simulink model "bldc_motor_controller_full_count"  (R2017a)
settings: Solver=FixedStepAuto  StartTime=0.0  StopTime=50000  FixedStep=1  RelTol=1e-3  EnableMultiTasking=on
libraries: simulink x10
settings Model: Creator=michael.cox4  LastModifiedBy=michael.cox4
settings OptimizationCC: DefaultParameterBehavior=Inlined  PassReuseOutputArgsAs=Individual arguments  MaxStackSize=64
settings DebuggingCC: ParameterTunabilityLossMsg=error
settings HardwareCC: ProdBitPerPointer=32  ProdBitPerSizeT=32  ProdBitPerPtrDiffT=32  ProdLargestAtomicInteger=Long  ProdLargestAtomicFloat=Double  ProdWordSize=32  ProdHWDeviceType=ARM Compatible->ARM Cortex
settings SFSimCC: MATLABDynamicMemAlloc=off
settings RTWCC: SystemTargetFile=ert.tlc  TemplateMakefile=ert_default_tmf  Description=Embedded Coder  GenerateReport=on  Toolchain=GNU Tools for ARM Embedded Processors  IncludeHyperlinkInReport=on  LaunchReport=on  GenerateTraceInfo=on  GenerateTraceReport=on  GenerateTraceReportSl=on  GenerateTraceReportSf=on  GenerateTraceReportEml=on
settings CodeAppCC: ForceParamTrailComments=on  IgnoreCustomStorageClasses=off  OperatorAnnotations=on  SimulinkDataObjDesc=on  SFDataObjDesc=on  MATLABFcnDesc=on  InsertBlockDesc=on  MATLABSourceComments=on
settings ERTTargetCC: CodeReplacementLibrary=ARM Cortex-M (Optimized)  ERTCustomFileTemplate=example_file_process.tlc

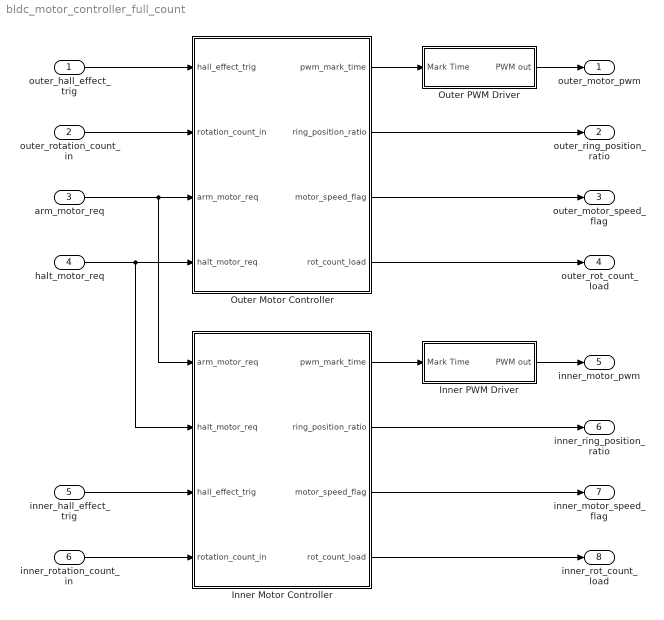
== system bldc_motor_controller_full_count ==
  outer_hall_effect_trig : Inport  OutDataTypeStr=boolean
  outer_rotation_count_in : Inport  Port=2
  arm_motor_req : Inport  Port=3
  halt_motor_req : Inport  Port=4
  inner_hall_effect_trig : Inport  Port=5  OutDataTypeStr=boolean
  inner_rotation_count_in : Inport  Port=6
  Inner Motor Controller : Subsystem
  Inner PWM Driver : Subsystem
  Outer Motor Controller : Subsystem
  Outer PWM Driver : Subsystem
  outer_motor_pwm : Outport
  outer_ring_position_ratio : Outport  Port=2
  outer_motor_speed_flag : Outport  Port=3
  outer_rot_count_load : Outport  Port=4
  inner_motor_pwm : Outport  Port=5
  inner_ring_position_ratio : Outport  Port=6
  inner_motor_speed_flag : Outport  Port=7
  inner_rot_count_load : Outport  Port=8
  wires:
  Outer Motor Controller/2(ring_position_ratio) -> outer_ring_position_ratio/1
  Outer Motor Controller/3(motor_speed_flag) -> outer_motor_speed_flag/1
  Outer PWM Driver/1(PWM out) -> outer_motor_pwm/1
  arm_motor_req/1 -> Outer Motor Controller/3(arm_motor_req), Inner Motor Controller/1(arm_motor_req)
  Outer Motor Controller/1(pwm_mark_time) -> Outer PWM Driver/1(Mark Time)
  outer_hall_effect_trig/1 -> Outer Motor Controller/1(hall_effect_trig)
  halt_motor_req/1 -> Outer Motor Controller/4(halt_motor_req), Inner Motor Controller/2(halt_motor_req)
  outer_rotation_count_in/1 -> Outer Motor Controller/2(rotation_count_in)
  Outer Motor Controller/4(rot_count_load) -> outer_rot_count_load/1
  Inner PWM Driver/1(PWM out) -> inner_motor_pwm/1
  Inner Motor Controller/4(rot_count_load) -> inner_rot_count_load/1
  Inner Motor Controller/3(motor_speed_flag) -> inner_motor_speed_flag/1
  Inner Motor Controller/2(ring_position_ratio) -> inner_ring_position_ratio/1
  Inner Motor Controller/1(pwm_mark_time) -> Inner PWM Driver/1(Mark Time)
  inner_rotation_count_in/1 -> Inner Motor Controller/4(rotation_count_in)
  inner_hall_effect_trig/1 -> Inner Motor Controller/3(hall_effect_trig)

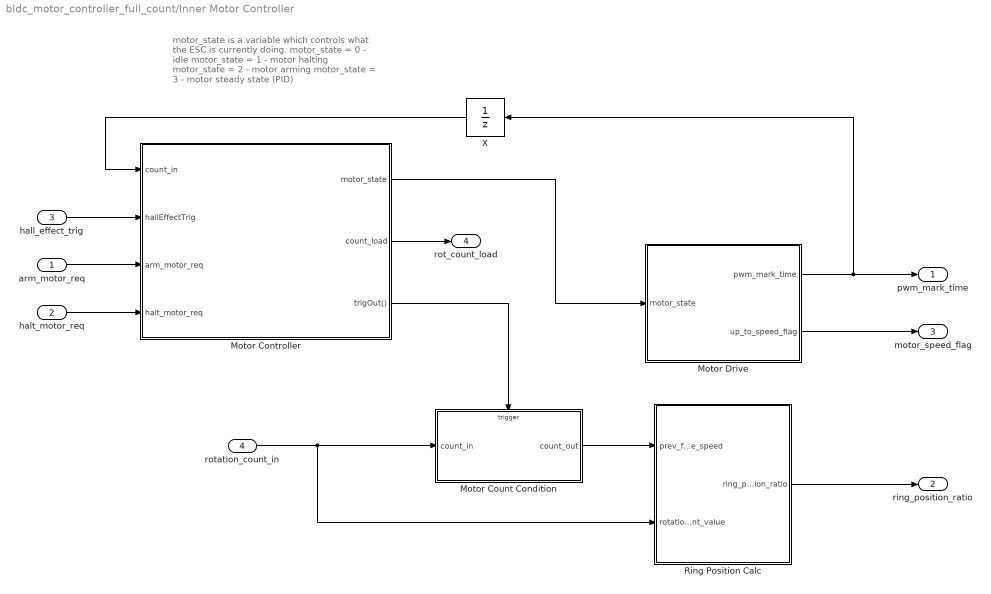
== system bldc_motor_controller_full_count/Inner Motor Controller ==
  note: motor_state is a variable which controls
      | what the ESC is currently doing.
      |   motor_state = 0 - idle
      |   motor_state = 1 - motor halting
      |   motor_state = 2 - motor arming
      |   motor_state = 3 - motor steady state (PID)
  arm_motor_req : Inport  OutDataTypeStr=boolean
  halt_motor_req : Inport  Port=2  OutDataTypeStr=boolean
  hall_effect_trig : Inport  Port=3  OutDataTypeStr=boolean
  rotation_count_in : Inport  Port=4
  Motor Controller : Stateflow chart  TreatAsAtomicUnit=on
  Motor Count Condition : Subsystem  TreatAsAtomicUnit=on
  Motor Drive : Subsystem
  Ring Position Calc : Subsystem
  X : UnitDelay  SampleTime=-1  StateName=X
  pwm_mark_time : Outport
  ring_position_ratio : Outport  Port=2
  motor_speed_flag : Outport  Port=3
  rot_count_load : Outport  Port=4
  wires:
  Motor Controller/3(trigOut()) -> Motor Count Condition/Trigger
  Motor Controller/2(count_load) -> rot_count_load/1
  Motor Count Condition/1(count_out) -> Ring Position Calc/1(prev_frame_speed)
  rotation_count_in/1 -> Motor Count Condition/1(count_in), Ring Position Calc/2(rotation_count_value)
  Motor Controller/1(motor_state) -> Motor Drive/1(motor_state)
  arm_motor_req/1 -> Motor Controller/3(arm_motor_req)
  halt_motor_req/1 -> Motor Controller/4(halt_motor_req)
  Ring Position Calc/1(ring_position_ratio) -> ring_position_ratio/1
  Motor Drive/1(pwm_mark_time) -> X/1, pwm_mark_time/1
  hall_effect_trig/1 -> Motor Controller/2(hallEffectTrig)
  X/1 -> Motor Controller/1(count_in)
  Motor Drive/2(up_to_speed_flag) -> motor_speed_flag/1

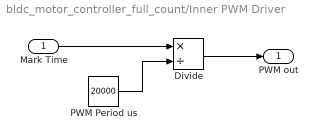
== system bldc_motor_controller_full_count/Inner PWM Driver ==
  Mark Time : Inport
  Divide : Product  Inputs=*/
  PWM Period us : Constant  Value=20000
  PWM out : Outport
  wires:
  Mark Time/1 -> Divide/1
  PWM Period us/1 -> Divide/2
  Divide/1 -> PWM out/1

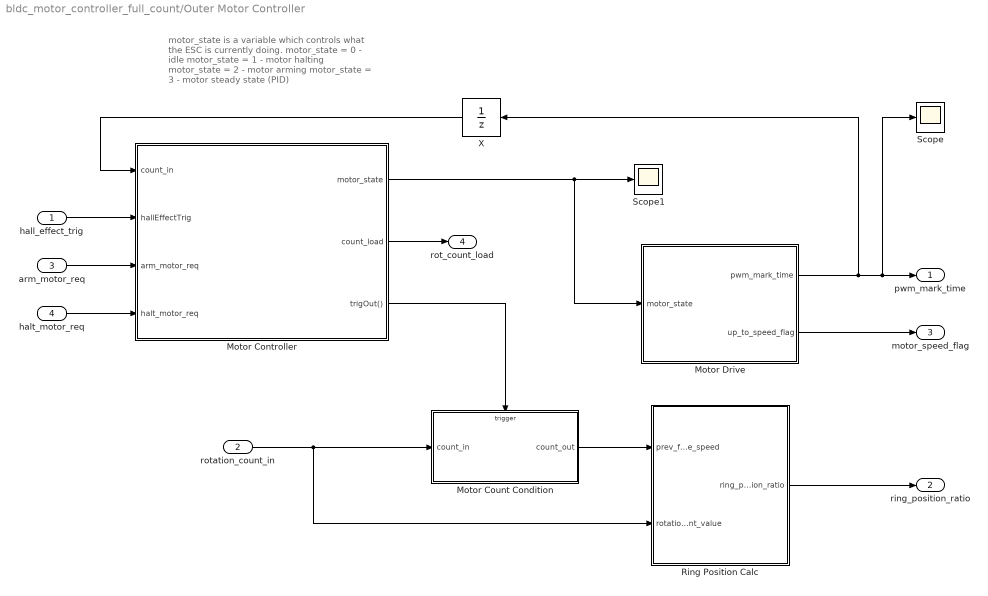
== system bldc_motor_controller_full_count/Outer Motor Controller ==
  note: motor_state is a variable which controls
      | what the ESC is currently doing.
      |   motor_state = 0 - idle
      |   motor_state = 1 - motor halting
      |   motor_state = 2 - motor arming
      |   motor_state = 3 - motor steady state (PID)
  hall_effect_trig : Inport  OutDataTypeStr=boolean
  rotation_count_in : Inport  Port=2
  arm_motor_req : Inport  Port=3  OutDataTypeStr=boolean
  halt_motor_req : Inport  Port=4  OutDataTypeStr=boolean
  Motor Controller : Stateflow chart  TreatAsAtomicUnit=on
  Motor Count Condition : Subsystem  TreatAsAtomicUnit=on
  Motor Drive : Subsystem
  Ring Position Calc : Subsystem
  Scope : Scope
  Scope1 : Scope
  X : UnitDelay  SampleTime=-1  StateName=X
  pwm_mark_time : Outport
  ring_position_ratio : Outport  Port=2
  motor_speed_flag : Outport  Port=3
  rot_count_load : Outport  Port=4
  wires:
  Motor Controller/3(trigOut()) -> Motor Count Condition/Trigger
  Motor Controller/2(count_load) -> rot_count_load/1
  Motor Count Condition/1(count_out) -> Ring Position Calc/1(prev_frame_speed)
  rotation_count_in/1 -> Motor Count Condition/1(count_in), Ring Position Calc/2(rotation_count_value)
  Motor Controller/1(motor_state) -> Scope1/1, Motor Drive/1(motor_state)
  Ring Position Calc/1(ring_position_ratio) -> ring_position_ratio/1
  Motor Drive/1(pwm_mark_time) -> X/1, Scope/1, pwm_mark_time/1
  X/1 -> Motor Controller/1(count_in)
  Motor Drive/2(up_to_speed_flag) -> motor_speed_flag/1
  hall_effect_trig/1 -> Motor Controller/2(hallEffectTrig)
  halt_motor_req/1 -> Motor Controller/4(halt_motor_req)
  arm_motor_req/1 -> Motor Controller/3(arm_motor_req)

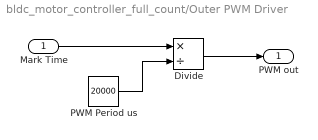
== system bldc_motor_controller_full_count/Outer PWM Driver ==
  Mark Time : Inport
  Divide : Product  Inputs=*/
  PWM Period us : Constant  Value=20000
  PWM out : Outport
  wires:
  Mark Time/1 -> Divide/1
  PWM Period us/1 -> Divide/2
  Divide/1 -> PWM out/1

== system bldc_motor_controller_full_count/Inner Motor Controller/Motor Count Condition ==
  count_in : Inport
  function : TriggerPort  TriggerType=function-call  VariantControl=Variant
  count_out : Outport
  wires:
  count_in/1 -> count_out/1

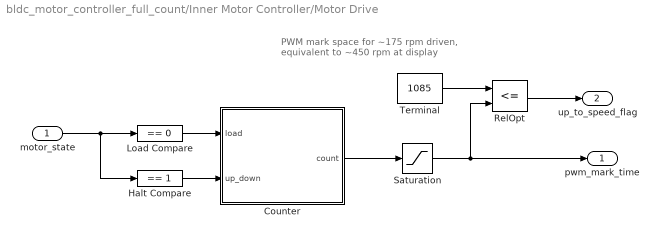
== system bldc_motor_controller_full_count/Inner Motor Controller/Motor Drive ==
  note: PWM mark space for ~175 rpm driven,
      | equivalent to ~450 rpm at display
  motor_state : Inport
  Counter : Subsystem
  Halt Compare : simulink/Logic and Bit Operations/Compare To Constant  relop===  const=1  OutDataTypeStr=boolean
  Load Compare : simulink/Logic and Bit Operations/Compare To Constant  relop===  const=0  OutDataTypeStr=boolean
  RelOpt : RelationalOperator  Operator=<=  OutDataTypeStr=boolean  RndMeth=Nearest  InputSameDT=on
  Saturation : Saturate  UpperLimit=1200  OutDataTypeStr=Inherit: Inherit via back propagation
  Terminal : Constant  Value=1085  OutDataTypeStr=Inherit: Inherit via back propagation
  pwm_mark_time : Outport
  up_to_speed_flag : Outport  Port=2
  wires:
  Counter/1(count) -> Saturation/1
  Terminal/1 -> RelOpt/1
  RelOpt/1 -> up_to_speed_flag/1
  Load Compare/1 -> Counter/1(load)
  Halt Compare/1 -> Counter/2(up_down)
  motor_state/1 -> Halt Compare/1, Load Compare/1
  Saturation/1 -> RelOpt/2, pwm_mark_time/1

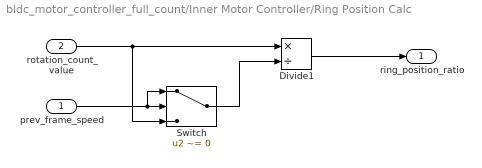
== system bldc_motor_controller_full_count/Inner Motor Controller/Ring Position Calc ==
  prev_frame_speed : Inport
  rotation_count_value : Inport  Port=2
  Divide1 : Product  Inputs=*/  OutDataTypeStr=single  RndMeth=Round
  Switch : Switch  Criteria=u2 ~= 0
  ring_position_ratio : Outport
  wires:
  rotation_count_value/1 -> Switch/3, Divide1/1
  Divide1/1 -> ring_position_ratio/1
  Switch/1 -> Divide1/2
  prev_frame_speed/1 -> Switch/1, Switch/2

== system bldc_motor_controller_full_count/Outer Motor Controller/Motor Count Condition ==
  count_in : Inport
  function : TriggerPort  TriggerType=function-call  VariantControl=Variant
  count_out : Outport
  wires:
  count_in/1 -> count_out/1

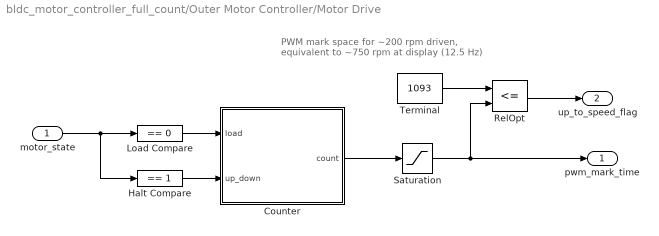
== system bldc_motor_controller_full_count/Outer Motor Controller/Motor Drive ==
  note: PWM mark space for ~200 rpm driven,
      | equivalent to ~750 rpm at display (12.5 Hz)
  motor_state : Inport
  Counter : Subsystem
  Halt Compare : simulink/Logic and Bit Operations/Compare To Constant  relop===  const=1  OutDataTypeStr=boolean
  Load Compare : simulink/Logic and Bit Operations/Compare To Constant  relop===  const=0  OutDataTypeStr=boolean
  RelOpt : RelationalOperator  Operator=<=  OutDataTypeStr=boolean  RndMeth=Nearest  InputSameDT=on
  Saturation : Saturate  UpperLimit=1250  OutDataTypeStr=Inherit: Inherit via back propagation
  Terminal : Constant  Value=1093  OutDataTypeStr=Inherit: Inherit via back propagation
  pwm_mark_time : Outport
  up_to_speed_flag : Outport  Port=2
  wires:
  Counter/1(count) -> Saturation/1
  Terminal/1 -> RelOpt/1
  RelOpt/1 -> up_to_speed_flag/1
  Load Compare/1 -> Counter/1(load)
  Halt Compare/1 -> Counter/2(up_down)
  motor_state/1 -> Halt Compare/1, Load Compare/1
  Saturation/1 -> RelOpt/2, pwm_mark_time/1

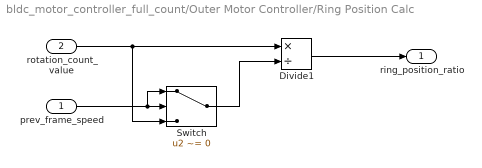
== system bldc_motor_controller_full_count/Outer Motor Controller/Ring Position Calc ==
  prev_frame_speed : Inport
  rotation_count_value : Inport  Port=2
  Divide1 : Product  Inputs=*/  OutDataTypeStr=single  RndMeth=Round
  Switch : Switch  Criteria=u2 ~= 0
  ring_position_ratio : Outport
  wires:
  rotation_count_value/1 -> Switch/3, Divide1/1
  Divide1/1 -> ring_position_ratio/1
  Switch/1 -> Divide1/2
  prev_frame_speed/1 -> Switch/1, Switch/2

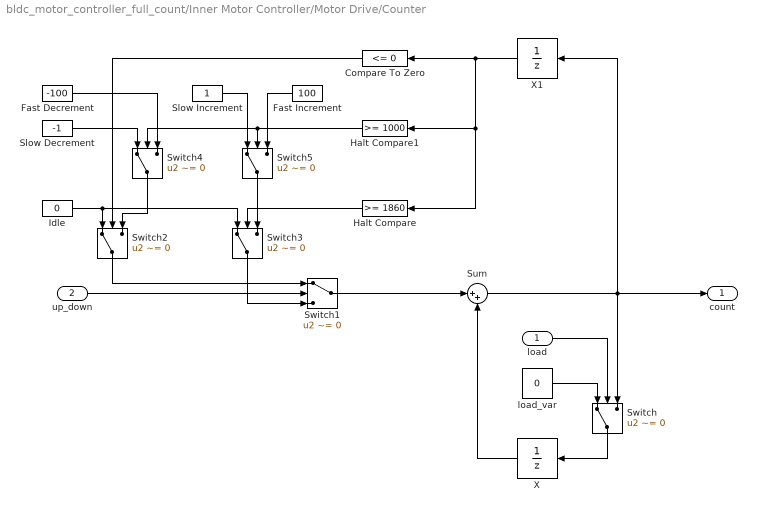
== system bldc_motor_controller_full_count/Inner Motor Controller/Motor Drive/Counter ==
  load : Inport
  up_down : Inport  Port=2
  Compare To Zero : simulink/Logic and Bit Operations/Compare To Zero  relop=<=  OutDataTypeStr=boolean
  Fast Decrement : Constant  Value=-100  OutDataTypeStr=Inherit: Inherit via back propagation
  Fast Increment : Constant  Value=100
  Halt Compare : simulink/Logic and Bit Operations/Compare To Constant  relop=>=  const=1860  OutDataTypeStr=boolean
  Halt Compare1 : simulink/Logic and Bit Operations/Compare To Constant  relop=>=  const=1000  OutDataTypeStr=boolean
  Idle : Constant  Value=0  OutDataTypeStr=Inherit: Inherit via back propagation
  Slow Decrement : Constant  Value=-1  OutDataTypeStr=Inherit: Inherit via back propagation
  Slow Increment : Constant
  Sum : Sum  Inputs=|++  OutMin=0  OutMax=1196  OutDataTypeStr=Inherit: Inherit via back propagation
  Switch{,2..5} (5 alike) : Switch  Criteria=u2 ~= 0  Threshold=.5  OutMax=1196  InputSameDT=on
  Switch1 : Switch  Criteria=u2 ~= 0  Threshold=.5  InputSameDT=on
  X : UnitDelay  SampleTime=-1  StateName=X
  X1 : UnitDelay  SampleTime=-1  StateName=X
  load_var : Constant  Value=0
  count : Outport
  wires:
  Sum/1 -> X1/1, Switch/3, count/1
  X/1 -> Sum/2
  Switch/1 -> X/1
  load/1 -> Switch/2
  load_var/1 -> Switch/1
  up_down/1 -> Switch1/2
  Switch1/1 -> Sum/1
  Switch2/1 -> Switch1/1
  Switch3/1 -> Switch1/3
  X1/1 -> Halt Compare/1, Halt Compare1/1, Compare To Zero/1
  Halt Compare/1 -> Switch3/2
  Compare To Zero/1 -> Switch2/2
  Idle/1 -> Switch2/1, Switch3/1
  Fast Decrement/1 -> Switch4/3
  Halt Compare1/1 -> Switch5/2, Switch4/2
  Switch4/1 -> Switch2/3
  Slow Decrement/1 -> Switch4/1
  Switch5/1 -> Switch3/3
  Slow Increment/1 -> Switch5/1
  Fast Increment/1 -> Switch5/3

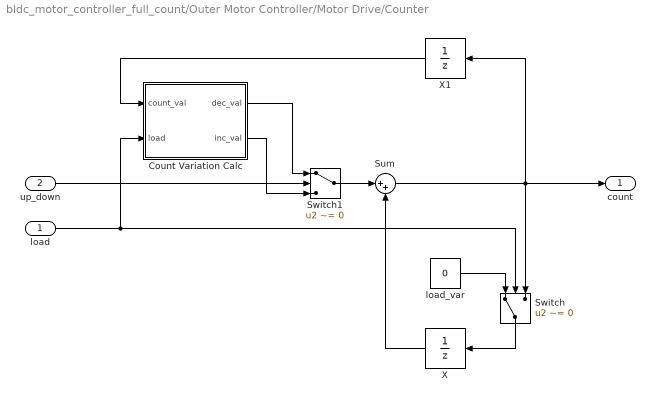
== system bldc_motor_controller_full_count/Outer Motor Controller/Motor Drive/Counter ==
  load : Inport
  up_down : Inport  Port=2
  Count Variation Calc : Subsystem
  Sum : Sum  Inputs=|++  OutMin=0  OutMax=1196  OutDataTypeStr=Inherit: Inherit via back propagation
  Switch : Switch  Criteria=u2 ~= 0  Threshold=.5  OutMax=1196  InputSameDT=on
  Switch1 : Switch  Criteria=u2 ~= 0  Threshold=.5  InputSameDT=on
  X : UnitDelay  SampleTime=-1  StateName=X
  X1 : UnitDelay  SampleTime=-1  StateName=X
  load_var : Constant  Value=0
  count : Outport
  wires:
  Sum/1 -> X1/1, Switch/3, count/1
  X/1 -> Sum/2
  Switch/1 -> X/1
  load_var/1 -> Switch/1
  up_down/1 -> Switch1/2
  Switch1/1 -> Sum/1
  Count Variation Calc/1(dec_val) -> Switch1/1
  X1/1 -> Count Variation Calc/1(count_val)
  load/1 -> Count Variation Calc/2(load), Switch/2
  Count Variation Calc/2(inc_val) -> Switch1/3

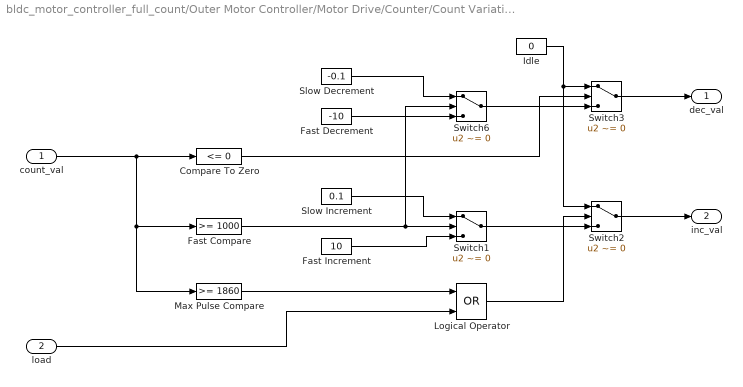
== system bldc_motor_controller_full_count/Outer Motor Controller/Motor Drive/Counter/Count Variation Calc ==
  count_val : Inport
  load : Inport  Port=2
  Compare To Zero : simulink/Logic and Bit Operations/Compare To Zero  relop=<=  OutDataTypeStr=boolean
  Fast Compare : simulink/Logic and Bit Operations/Compare To Constant  relop=>=  const=1000  OutDataTypeStr=boolean
  Fast Decrement : Constant  Value=-10  OutDataTypeStr=Inherit: Inherit via back propagation
  Fast Increment : Constant  Value=10
  Idle : Constant  Value=0  OutDataTypeStr=Inherit: Inherit via back propagation
  Logical Operator : Logic  Operator=OR  AllPortsSameDT=off  OutDataTypeStr=boolean
  Max Pulse Compare : simulink/Logic and Bit Operations/Compare To Constant  relop=>=  const=1860  OutDataTypeStr=boolean
  Slow Decrement : Constant  Value=-0.1  OutDataTypeStr=Inherit: Inherit via back propagation
  Slow Increment : Constant  Value=0.1
  Switch{1..3,6} (4 alike) : Switch  Criteria=u2 ~= 0  Threshold=.5  OutMax=1196  InputSameDT=on
  dec_val : Outport
  inc_val : Outport  Port=2
  wires:
  load/1 -> Logical Operator/2
  Max Pulse Compare/1 -> Logical Operator/1
  Fast Compare/1 -> Switch6/2, Switch1/2
  Fast Decrement/1 -> Switch6/3
  Slow Decrement/1 -> Switch6/1
  Slow Increment/1 -> Switch1/1
  Fast Increment/1 -> Switch1/3
  count_val/1 -> Compare To Zero/1, Max Pulse Compare/1, Fast Compare/1
  Logical Operator/1 -> Switch2/2
  Switch1/1 -> Switch2/3
  Switch6/1 -> Switch3/3
  Idle/1 -> Switch3/1, Switch2/1
  Switch2/1 -> inc_val/1
  Switch3/1 -> dec_val/1
  Compare To Zero/1 -> Switch3/2

== stateflow chart bldc_motor_controller_full_count/Inner Motor Controller/Motor Controller ==
  settings: sampleTime=0
  state arm_motor [group]
    state idle
      entry:
      count_load = true;
      motor_state = 0;
    state arm_motor
      entry: motor_state = 2;
    (default) -> idle
    idle -> arm_motor.arm_motor : [arm_motor_req == 1]
  note: motor_state = 0 - idle
      |   motor_state = 1 - motor halting
      |   motor_state = 2 - motor arming
      |   motor_state = 3 - motor steady state (PID)
  state motor_ctrl_loop [group]
    state trig_idle
      entry:
      motor_state = 3;
      count_load = false;
    state speed_calc_done
      entry: count_load = true;
    state interrupt_trigger
      entry: trigOut;
    speed_calc_done -> trig_idle
    trig_idle -> interrupt_trigger [order 2] : [hallEffectTrig]
    interrupt_trigger -> speed_calc_done
  state halt_motor [group]
    state halt_motor
      entry:
      motor_state = 1;
  halt_motor.halt_motor -> idle : [halt_motor_req == 0 && count_in <= 1060]
  arm_motor.arm_motor -> trig_idle : [hallEffectTrig]
  trig_idle -> halt_motor.halt_motor [order 1] : [halt_motor_req == 1]
  data: count_in input; motor_state output uint8; hallEffectTrig input boolean; arm_motor_req input boolean; halt_motor_req input boolean; count_load output boolean
  events: trigOut output FUNCTION_CALL_EVENT

== stateflow chart bldc_motor_controller_full_count/Outer Motor Controller/Motor Controller ==
  settings: sampleTime=0
  state arm_motor [group]
    state idle
      entry:
      count_load = true;
      motor_state = 0;
    state arm_motor
      entry: motor_state = 2;
    (default) -> idle
    idle -> arm_motor.arm_motor : [arm_motor_req == 1]
  note: motor_state = 0 - idle
      |   motor_state = 1 - motor halting
      |   motor_state = 2 - motor arming
      |   motor_state = 3 - motor steady state (PID)
  state motor_ctrl_loop [group]
    state trig_idle
      entry:
      motor_state = 3;
      count_load = false;
    state speed_calc_done
      entry: count_load = true;
    state interrupt_trigger
      entry: trigOut;
    speed_calc_done -> trig_idle
    trig_idle -> interrupt_trigger [order 2] : [hallEffectTrig]
    interrupt_trigger -> speed_calc_done
  state halt_motor [group]
    state halt_motor
      entry:
      motor_state = 1;
  halt_motor.halt_motor -> idle : [halt_motor_req == 0 && count_in <= 0]
  arm_motor.arm_motor -> trig_idle : [hallEffectTrig]
  trig_idle -> halt_motor.halt_motor [order 1] : [halt_motor_req == 1]
  data: count_in input; motor_state output uint8; hallEffectTrig input boolean; arm_motor_req input boolean; halt_motor_req input boolean; count_load output boolean
  events: trigOut output FUNCTION_CALL_EVENT
